simulink model "Ejercicio10_13_02_17"  (R2013a)
settings: Solver=ode45  StartTime=0.0  StopTime=10.0  RelTol=1e-3
settings Model: Creator=Miguel  LastModifiedBy=Miguel

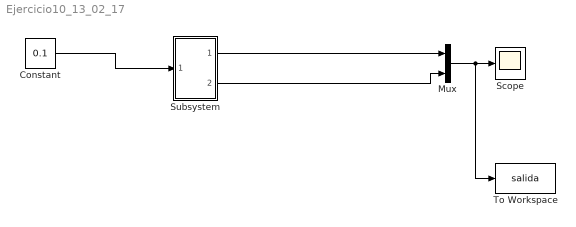
== system Ejercicio10_13_02_17 ==
  Constant : Constant  Value=0.1
  Mux : Mux  Inputs=2
  Scope : Scope
      settings: ShowLegends=on
  Subsystem : Subsystem
  To Workspace : ToWorkspace  VariableName=salida  SampleTime=-1
  wires:
  Mux/1 -> To Workspace/1, Scope/1
  Constant/1 -> Subsystem/1(In1)
  Subsystem/1(Out1) -> Mux/1
  Subsystem/2(Out2) -> Mux/2

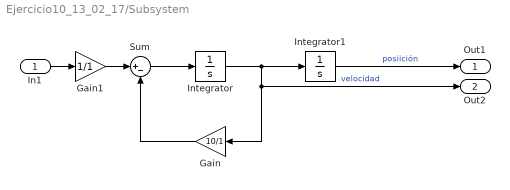
== system Ejercicio10_13_02_17/Subsystem ==
  In1 : Inport
  Gain : Gain  Gain=10/1
  Gain1 : Gain  Gain=1/1
  Integrator : Integrator  InitialCondition=-1
  Integrator1 : Integrator
  Sum : Sum  Inputs=|+-
  Out1 : Outport
  Out2 : Outport  Port=2
  wires:
  Gain1/1 -> Sum/1
  Integrator/1 -> Gain/1, Out2/1, Integrator1/1  "velocidad"
  Sum/1 -> Integrator/1
  Integrator1/1 -> Out1/1  "posiición"
  Gain/1 -> Sum/2
  In1/1 -> Gain1/1
